simulink subsystem "GUIDANCE_MSG_UNMAP"  (R2023a)
settings: Solver=VariableStepAuto  StartTime=0.0  StopTime=10.0  RelTol=1e-3
libraries: sharedtransform x1
settings Model: Creator=thesa  LastModifiedBy=thesa

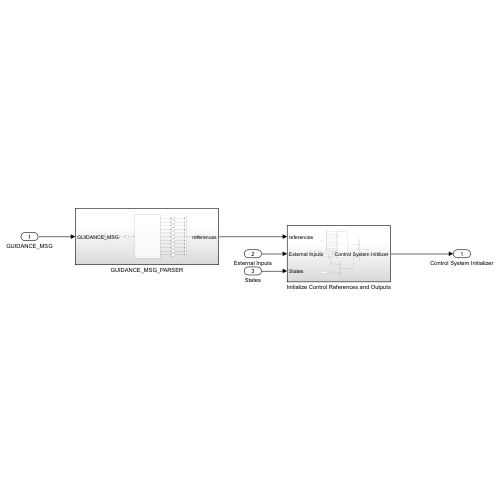
[thumbnail: Simulink's stored preview of the top-level diagram]
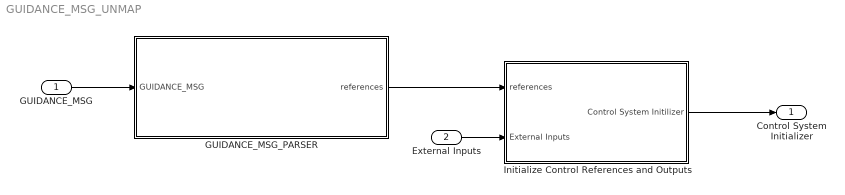
== system GUIDANCE_MSG_UNMAP ==
  GUIDANCE_MSG : Inport
  External Inputs : Inport  Port=2
  GUIDANCE_MSG_PARSER : Subsystem
  Initialize Control References and Outputs : Subsystem
  Control System Initializer : Outport
  wires:
  External Inputs/1 -> Initialize Control References and Outputs/2(External Inputs)
  GUIDANCE_MSG_PARSER/1(references) -> Initialize Control References and Outputs/1(references)
  GUIDANCE_MSG/1 -> GUIDANCE_MSG_PARSER/1(GUIDANCE_MSG)
  Initialize Control References and Outputs/1(Control System Initilizer) -> Control System Initializer/1

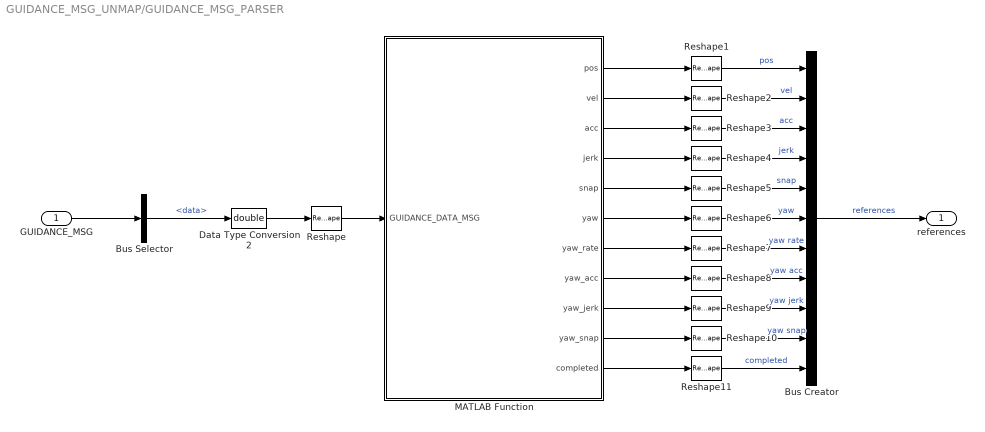
== system GUIDANCE_MSG_UNMAP/GUIDANCE_MSG_PARSER ==
  GUIDANCE_MSG : Inport
  Bus Creator : BusCreator  Inputs=11
  Bus Selector : BusSelector  OutputSignals=data
  Data Type Conversion2 : DataTypeConversion  OutDataTypeStr=double  SaturateOnIntegerOverflow=off  RndMeth=Floor
  MATLAB Function : MATLAB Function  TreatAsAtomicUnit=on
  Reshape{,1..11} (12 alike) : Reshape
  references : Outport
  wires:
  Reshape/1 -> MATLAB Function/1(GUIDANCE_DATA_MSG)
  GUIDANCE_MSG/1 -> Bus Selector/1
  Data Type Conversion2/1 -> Reshape/1
  Bus Selector/1 -> Data Type Conversion2/1  "<data>"
  Bus Creator/1 -> references/1  "references"
  Reshape1/1 -> Bus Creator/1  "pos"
  Reshape2/1 -> Bus Creator/2  "vel"
  Reshape3/1 -> Bus Creator/3  "acc"
  Reshape4/1 -> Bus Creator/4  "jerk"
  Reshape5/1 -> Bus Creator/5  "snap"
  Reshape6/1 -> Bus Creator/6  "yaw"
  Reshape7/1 -> Bus Creator/7  "yaw rate"
  Reshape8/1 -> Bus Creator/8  "yaw acc"
  Reshape9/1 -> Bus Creator/9  "yaw jerk"
  Reshape10/1 -> Bus Creator/10  "yaw snap"
  MATLAB Function/1(pos) -> Reshape1/1
  MATLAB Function/2(vel) -> Reshape2/1
  MATLAB Function/3(acc) -> Reshape3/1
  MATLAB Function/4(jerk) -> Reshape4/1
  MATLAB Function/5(snap) -> Reshape5/1
  MATLAB Function/6(yaw) -> Reshape6/1
  MATLAB Function/7(yaw_rate) -> Reshape7/1
  MATLAB Function/8(yaw_acc) -> Reshape8/1
  MATLAB Function/9(yaw_jerk) -> Reshape9/1
  MATLAB Function/10(yaw_snap) -> Reshape10/1
  MATLAB Function/11(completed) -> Reshape11/1
  Reshape11/1 -> Bus Creator/11  "completed"

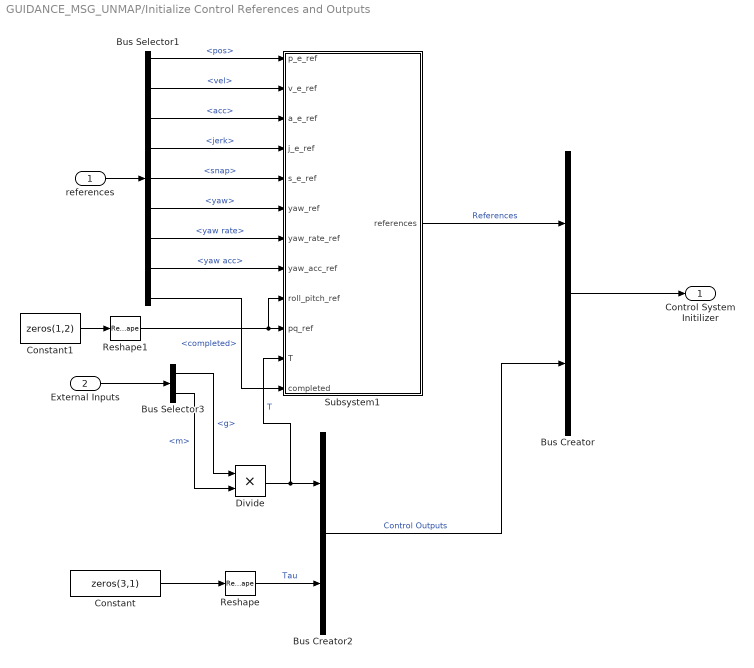
== system GUIDANCE_MSG_UNMAP/Initialize Control References and Outputs ==
  references : Inport
  External Inputs : Inport  Port=2
  Bus Creator : BusCreator  Inputs=2
  Bus Creator2 : BusCreator  Inputs=2
  Bus Selector1 : BusSelector  OutputSignals=pos,vel,acc,jerk,snap,yaw,yaw rate,yaw acc,completed
  Bus Selector3 : BusSelector  OutputSignals=Vehicle Parameters.g,Vehicle Parameters.m
  Constant : Constant  Value=zeros(3,1)
  Constant1 : Constant  Value=zeros(1,2)
  Divide : Product  Inputs=**
  Reshape : Reshape  OutputDimensionality=Column vector (2-D)
  Reshape1 : Reshape
  Subsystem1 : Subsystem
  Control System Initilizer : Outport
  wires:
  Constant1/1 -> Reshape1/1
  Subsystem1/1(references) -> Bus Creator/1  "References"
  references/1 -> Bus Selector1/1
  Bus Selector3/1 -> Divide/1  "<g>"
  External Inputs/1 -> Bus Selector3/1
  Bus Creator/1 -> Control System Initilizer/1
  Divide/1 -> Bus Creator2/1, Subsystem1/11(T)  "T"
  Constant/1 -> Reshape/1
  Bus Creator2/1 -> Bus Creator/2  "Control Outputs"
  Reshape/1 -> Bus Creator2/2  "Tau"
  Bus Selector3/2 -> Divide/2  "<m>"
  Bus Selector1/1 -> Subsystem1/1(p_e_ref)  "<pos>"
  Bus Selector1/2 -> Subsystem1/2(v_e_ref)  "<vel>"
  Bus Selector1/3 -> Subsystem1/3(a_e_ref)  "<acc>"
  Bus Selector1/4 -> Subsystem1/4(j_e_ref)  "<jerk>"
  Bus Selector1/5 -> Subsystem1/5(s_e_ref)  "<snap>"
  Bus Selector1/6 -> Subsystem1/6(yaw_ref)  "<yaw>"
  Bus Selector1/7 -> Subsystem1/7(yaw_rate_ref)  "<yaw rate>"
  Bus Selector1/8 -> Subsystem1/8(yaw_acc_ref)  "<yaw acc>"
  Reshape1/1 -> Subsystem1/10(pq_ref), Subsystem1/9(roll_pitch_ref)
  Bus Selector1/9 -> Subsystem1/12(completed)  "<completed>"

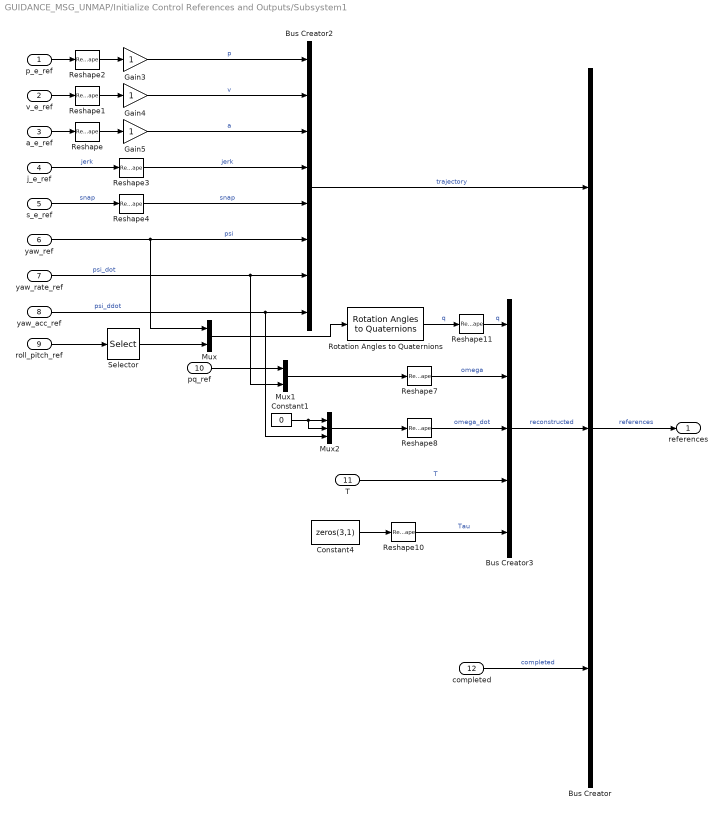
== system GUIDANCE_MSG_UNMAP/Initialize Control References and Outputs/Subsystem1 ==
  p_e_ref : Inport
  v_e_ref : Inport  Port=2
  a_e_ref : Inport  Port=3
  j_e_ref : Inport  Port=4
  s_e_ref : Inport  Port=5
  yaw_ref : Inport  Port=6
  yaw_rate_ref : Inport  Port=7
  yaw_acc_ref : Inport  Port=8
  roll_pitch_ref : Inport  Port=9
  pq_ref : Inport  Port=10
  T : Inport  Port=11
  completed : Inport  Port=12
  Bus Creator : BusCreator  Inputs=3
  Bus Creator2 : BusCreator  Inputs=8
  Bus Creator3 : BusCreator  Inputs=5
  Constant1 : Constant  Value=0
  Constant4 : Constant  Value=zeros(3,1)
  Gain3 : Gain
  Gain4 : Gain
  Gain5 : Gain
  Mux : Mux  Inputs=2
  Mux1 : Mux  Inputs=2
  Mux2 : Mux  Inputs=3
  Reshape{,1..4,7..8,10} (8 alike) : Reshape  OutputDimensionality=Column vector (2-D)
  Reshape11 : Reshape  OutputDimensionality=Row vector (2-D)
  Rotation Angles to Quaternions : sharedtransform/Rotation Angles to Quaternions  rotationOrder=ZYX  aMode=aMode
  Selector : Selector  InputPortWidth=2  IndexOptions=Index vector (dialog)  Indices=[2 1]  OutputSizes=1
  references : Outport
  wires:
  Reshape4/1 -> Bus Creator2/5  "snap"
  Reshape3/1 -> Bus Creator2/4  "jerk"
  Reshape2/1 -> Gain3/1
  Reshape1/1 -> Gain4/1
  Reshape/1 -> Gain5/1
  p_e_ref/1 -> Reshape2/1
  Gain3/1 -> Bus Creator2/1  "p"
  Gain5/1 -> Bus Creator2/3  "a"
  j_e_ref/1 -> Reshape3/1  "jerk"
  s_e_ref/1 -> Reshape4/1  "snap"
  yaw_ref/1 -> Bus Creator2/6, Mux/1  "psi"
  Gain4/1 -> Bus Creator2/2  "v"
  yaw_rate_ref/1 -> Mux1/2, Bus Creator2/7  "psi_dot"
  yaw_acc_ref/1 -> Mux2/3, Bus Creator2/8  "psi_ddot"
  Constant4/1 -> Reshape10/1
  pq_ref/1 -> Mux1/1
  Bus Creator/1 -> references/1  "references"
  T/1 -> Bus Creator3/4  "T"
  Reshape7/1 -> Bus Creator3/2  "omega"
  Rotation Angles to Quaternions/1 -> Reshape11/1  "q"
  Reshape8/1 -> Bus Creator3/3  "omega_dot"
  Reshape11/1 -> Bus Creator3/1  "q"
  v_e_ref/1 -> Reshape1/1
  a_e_ref/1 -> Reshape/1
  Bus Creator3/1 -> Bus Creator/2  "reconstructed"
  Bus Creator2/1 -> Bus Creator/1  "trajectory"
  Mux2/1 -> Reshape8/1
  Reshape10/1 -> Bus Creator3/5  "Tau"
  Mux/1 -> Rotation Angles to Quaternions/1
  roll_pitch_ref/1 -> Selector/1
  Selector/1 -> Mux/2
  Mux1/1 -> Reshape7/1
  Constant1/1 -> Mux2/2, Mux2/1
  completed/1 -> Bus Creator/3  "completed"

== matlab function GUIDANCE_MSG_UNMAP/GUIDANCE_MSG_PARSER/MATLAB Function ==
  data: GUIDANCE_DATA_MSG input; pos output; vel output; acc output; jerk output; snap output; yaw output; yaw_rate output; yaw_acc output; yaw_jerk output; yaw_snap output; completed output
function [pos, vel, acc, jerk, snap,...
    yaw, yaw_rate, yaw_acc, yaw_jerk, yaw_snap, completed]  = ...
    translation_guidance2ref(GUIDANCE_DATA_MSG)
N_DOFS = 4; %max number of dofs considered [x y z yaw]
pos_ = zeros(N_DOFS,1);
vel_ = zeros(N_DOFS,1);
acc_ = zeros(N_DOFS,1);
jerk_ = zeros(N_DOFS,1);
snap_ = zeros(N_DOFS,1);

pos = zeros(3,1);
vel = zeros(3,1);
acc = zeros(3,1);
jerk = zeros(3,1);
snap = zeros(3,1);
yaw = 0;
yaw_rate = 0; 
yaw_acc = 0; 
yaw_jerk = 0; 
yaw_snap = 0;
completed = false;

ind = 0;
ind = ind+1;
completed(1) = GUIDANCE_DATA_MSG(ind) > 0.2;

for i = 1:N_DOFS
    ind = ind + 1;
    pos_(i) = GUIDANCE_DATA_MSG(ind);
end
for i = 1:N_DOFS
    ind = ind + 1;
    vel_(i) = GUIDANCE_DATA_MSG(ind);
end
for i = 1:N_DOFS
    ind = ind + 1;
    acc_(i) = GUIDANCE_DATA_MSG(ind);
end
for i = 1:N_DOFS
    ind = ind + 1;
    jerk_(i) = GUIDANCE_DATA_MSG(ind);
end
for i = 1:N_DOFS
    ind = ind + 1;
    snap_(i) = GUIDANCE_DATA_MSG(ind);
end

if (N_DOFS > 3)
    for i = 1:3
        pos(i) = pos_(i);
        vel(i) = vel_(i);
        acc(i) = acc_(i);
        jerk(i) = jerk_(i);
        snap(i) = snap_(i);
    end
    yaw = pos_(4);
    yaw_rate = vel_(4); 
    yaw_acc = acc_(4); 
    yaw_jerk = jerk_(4); 
    yaw_snap = snap_(4);
else
    for i = 1:N_DOFS
        pos(i) = pos_(i);
        vel(i) = vel_(i);
        acc(i) = acc_(i);
        jerk(i) = jerk_(i);
        snap(i) = snap_(i);
    end
end

end
